simulink model "simulado"  (R2024a)
settings: Solver=VariableStepAuto  StartTime=0.0  StopTime=1.4  MaxStep=0.0001  RelTol=1e-3
values from neighbouring files (symbols this model uses):
  A = [0 1 0 0 0 0 ... (first row only)    [TP2.m]
  B = [0 0 0 ... (first row only)    [TP2.m]
  C = [1 0 0 0 0 0 ... (first row only)    [TP2.m]
  D = [0 0 0 ... (first row only)    [TP2.m]
  L = (place(A', C', polesObservateur))'    [TP2.m]
settings Model: Creator=vinicius.rocha-miran  LastModifiedBy=vinicius.rocha-miran

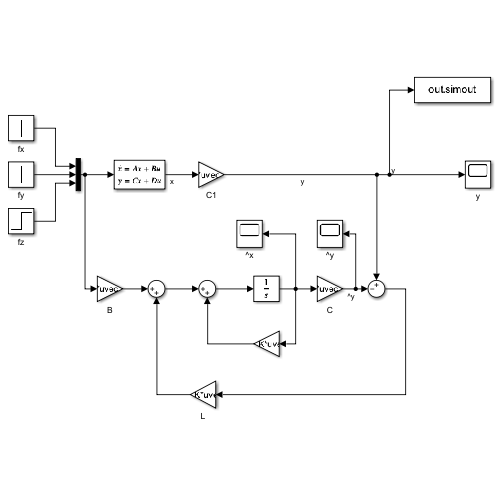
[thumbnail: Simulink's stored preview of the top-level diagram]
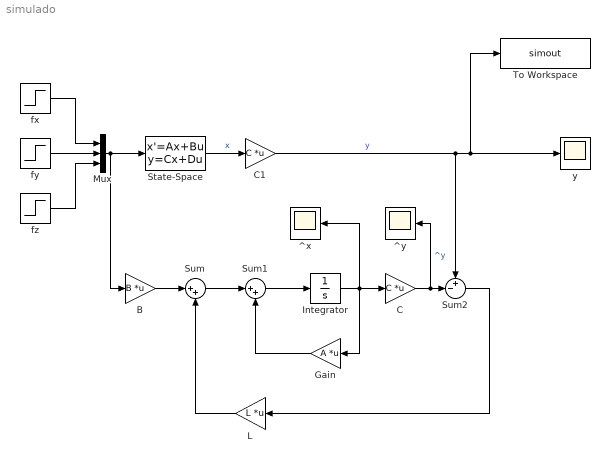
== system simulado ==
  B : Gain  Gain=B  Multiplication=Matrix(K*u) (u vector)
  C : Gain  Gain=C  Multiplication=Matrix(K*u) (u vector)
  C1 : Gain  Gain=C  Multiplication=Matrix(K*u) (u vector)
  Gain : Gain  Gain=A  Multiplication=Matrix(K*u) (u vector)
  Integrator : Integrator
  L : Gain  Gain=L  Multiplication=Matrix(K*u) (u vector)
  Mux : Mux  Inputs=3
  State-Space : StateSpace  A=A  B=B  C=C  D=D  InitialCondition=[0.1; 0; 0.1; 0; -0.1; 0]
  Sum : Sum  Inputs=|++
  Sum1 : Sum  Inputs=|++
  Sum2 : Sum  Inputs=+-|
  To Workspace : ToWorkspace  VariableName=simout  SaveFormat=Structure With Time  SampleTime=-1
  ^x : Scope
  ^y : Scope
  fx : Step  Before=1  SampleTime=0
  fy : Step  Before=1  SampleTime=0
  fz : Step  Before=1  SampleTime=0
  y : Scope
  wires:
  fx/1 -> Mux/1
  fy/1 -> Mux/2
  fz/1 -> Mux/3
  Mux/1 -> B/1, State-Space/1
  State-Space/1 -> C1/1  "x"
  B/1 -> Sum/1
  L/1 -> Sum/2
  Sum/1 -> Sum1/1
  Sum1/1 -> Integrator/1
  Integrator/1 -> ^x/1, Gain/1, C/1
  Gain/1 -> Sum1/2
  C/1 -> ^y/1, Sum2/2  "^y"
  Sum2/1 -> L/1
  C1/1 -> Sum2/1, To Workspace/1, y/1  "y"
